simulink model "ObstacleDetectionDemo"  (R2020a)
settings: Solver=FixedStepDiscrete  StartTime=0.0  StopTime=inf  FixedStep=params.Ts  RelTol=1e-3  EnableMultiTasking=on
PreLoadFcn:
  | params = controlParamsGazebo;
  | 
  | rosshutdown;
  | loadIpAddresses;
  | rosinit(gazeboIp);
model workspace (MAT data in the model file):
  SL_ROS_VariableLengthArrays_MaxSizes.CommonInfo.ArrayTruncateAction = 'EmitWarning'
  SL_ROS_VariableLengthArrays_MaxSizes.MsgTypeMap = containers.Map
  SL_ROS_VariableLengthArrays_MaxSizes.MsgTypeMap.serialization.keys = {'sensor_msgs/CompressedImage', 'sensor_msgs/Image'}
  SL_ROS_VariableLengthArrays_MaxSizes.MsgTypeMap.serialization.values{1}(1).PropertyName = 'Data'
  SL_ROS_VariableLengthArrays_MaxSizes.MsgTypeMap.serialization.values{1}(1).DataType = 'uint8'
  SL_ROS_VariableLengthArrays_MaxSizes.MsgTypeMap.serialization.values{1}(1).MaxLength = 26264
  SL_ROS_VariableLengthArrays_MaxSizes.MsgTypeMap.serialization.values{1}(2).PropertyName = 'Format'
  SL_ROS_VariableLengthArrays_MaxSizes.MsgTypeMap.serialization.values{1}(2).DataType = 'uint8'
  SL_ROS_VariableLengthArrays_MaxSizes.MsgTypeMap.serialization.values{1}(2).MaxLength = 128
  SL_ROS_VariableLengthArrays_MaxSizes.MsgTypeMap.serialization.values{2}(1).PropertyName = 'Data'
  SL_ROS_VariableLengthArrays_MaxSizes.MsgTypeMap.serialization.values{2}(1).DataType = 'uint8'
  SL_ROS_VariableLengthArrays_MaxSizes.MsgTypeMap.serialization.values{2}(1).MaxLength = 921600
  SL_ROS_VariableLengthArrays_MaxSizes.MsgTypeMap.serialization.values{2}(2).PropertyName = 'Encoding'
  SL_ROS_VariableLengthArrays_MaxSizes.MsgTypeMap.serialization.values{2}(2).DataType = 'uint8'
  SL_ROS_VariableLengthArrays_MaxSizes.MsgTypeMap.serialization.values{2}(2).MaxLength = 128
  SL_ROS_VariableLengthArrays_MaxSizes.MsgTypeMap.serialization.uniformity = 0
  SL_ROS_VariableLengthArrays_MaxSizes.MsgTypeMap.serialization.keyType = 'char'
  SL_ROS_VariableLengthArrays_MaxSizes.MsgTypeMap.serialization.valueType = 'any'
libraries: robotlib x11
settings Model: Creator=scastro  LastModifiedBy=shiva
settings SolverCC: PositivePriorityOrder=on
settings DataIOCC: ReturnWorkspaceOutputs=off
settings OptimizationCC: PassReuseOutputArgsAs=Individual arguments  MaxStackSize=64  EfficientTunableParamExpr=on
settings DebuggingCC: ParameterTunabilityLossMsg=error  ArithmeticOperatorsInVariantConditions=warning
settings HardwareCC: ProdBitPerLong=64  ProdHWDeviceType=Intel->x86-64 (Linux 64)  UseEmbeddedCoderFeatures=off
settings SFSimCC: SimUseLocalCustomCode=off  CustomCodeUndefinedFunction=UseInterfaceOnly
settings RTWCC: SystemTargetFile=ert.tlc  HardwareBoard=Robot Operating System (ROS)  TemplateMakefile=ert_default_tmf  GenerateReport=on  RTWUseLocalCustomCode=off  Toolchain=Catkin  IncludeHyperlinkInReport=on  LaunchReport=on  TargetLang=C++  GenerateTraceInfo=on  GenerateTraceReport=on  GenerateTraceReportSl=on  GenerateTraceReportSf=on  GenerateTraceReportEml=on
settings CodeAppCC: ForceParamTrailComments=on  IgnoreCustomStorageClasses=off  OperatorAnnotations=on  SimulinkDataObjDesc=on  SFDataObjDesc=on  MATLABFcnDesc=on  InsertBlockDesc=on  StateflowObjectComments=on  MATLABSourceComments=on
settings ERTTargetCC: SupportNonInlinedSFcns=on  SupportVariableSizeSignals=on

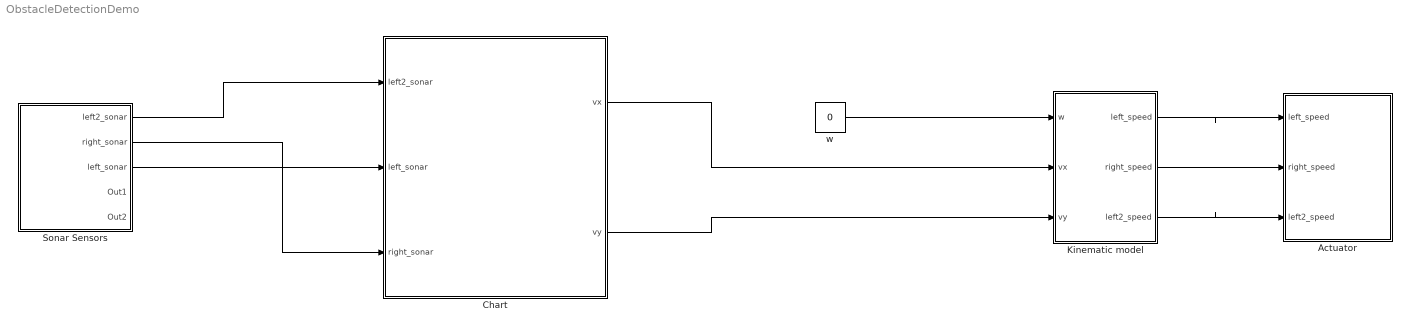
== system ObstacleDetectionDemo ==
  Actuator : Subsystem
  Chart : Stateflow chart  TreatAsAtomicUnit=on
  Kinematic model : Subsystem
  Sonar Sensors : Subsystem
  w : Constant  Value=0
  wires:
  w/1 -> Kinematic model/1(w)
  Chart/1(vx) -> Kinematic model/2(vx)
  Chart/2(vy) -> Kinematic model/3(vy)
  Kinematic model/1(left_speed) -> Actuator/1(left_speed)
  Kinematic model/2(right_speed) -> Actuator/2(right_speed)
  Kinematic model/3(left2_speed) -> Actuator/3(left2_speed)
  Sonar Sensors/1(left2_sonar) -> Chart/1(left2_sonar)
  Sonar Sensors/2(right_sonar) -> Chart/3(right_sonar)
  Sonar Sensors/3(left_sonar) -> Chart/2(left_sonar)

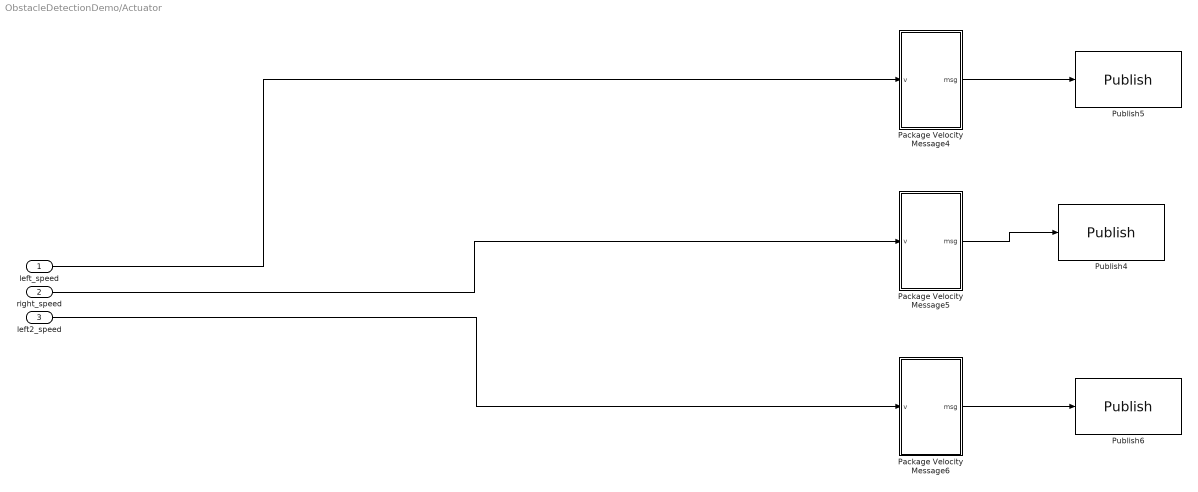
== system ObstacleDetectionDemo/Actuator ==
  left_speed : Inport
  right_speed : Inport  Port=2
  left2_speed : Inport  Port=3
  Package Velocity Message4 : Subsystem
  Package Velocity Message5 : Subsystem
  Package Velocity Message6 : Subsystem
  Publish4 : robotlib/Publish  topicSource=Select from ROS network  topic=/robot/right_joint_velocity_controller/command  messageType=std_msgs/Float64  messageQueueLength=1
  Publish5 : robotlib/Publish  topicSource=Select from ROS network  topic=/robot/left_joint_velocity_controller/command  messageType=std_msgs/Float64  messageQueueLength=1
  Publish6 : robotlib/Publish  topicSource=Select from ROS network  topic=/robot/left2_joint_velocity_controller/command  messageType=std_msgs/Float64  messageQueueLength=1
  wires:
  left_speed/1 -> Package Velocity Message4/1(v)
  Package Velocity Message6/1(msg) -> Publish6/1
  right_speed/1 -> Package Velocity Message5/1(v)
  Package Velocity Message4/1(msg) -> Publish5/1
  Package Velocity Message5/1(msg) -> Publish4/1
  left2_speed/1 -> Package Velocity Message6/1(v)

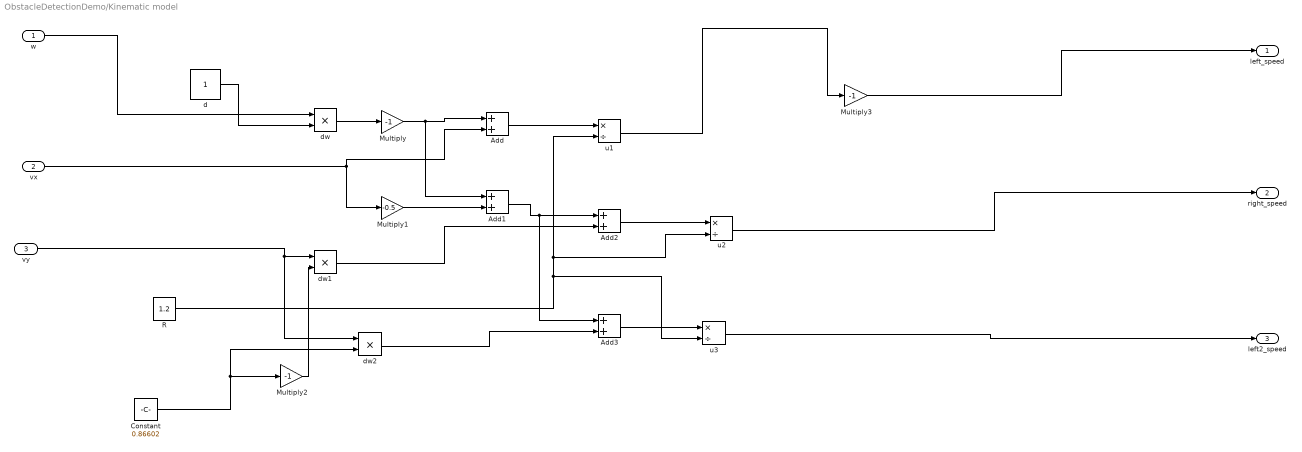
== system ObstacleDetectionDemo/Kinematic model ==
  w : Inport
  vx : Inport  Port=2
  vy : Inport  Port=3
  Add{,1..3} (4 alike) : Sum
  Constant : Constant  Value=0.86602
  Multiply : Gain  Gain=-1
  Multiply1 : Gain  Gain=-0.5
  Multiply2 : Gain  Gain=-1
  Multiply3 : Gain  Gain=-1
  R : Constant  Value=1.2
  d : Constant  VectorParams1D=off  SampleTime=-1
  dw : Product
  dw1 : Product
  dw2 : Product
  u1 : Product  Inputs=*/
  u2 : Product  Inputs=*/
  u3 : Product  Inputs=*/
  left_speed : Outport
  right_speed : Outport  Port=2
  left2_speed : Outport  Port=3
  wires:
  Multiply/1 -> Add1/1, Add/1
  Add/1 -> u1/1
  Multiply3/1 -> left_speed/1
  dw1/1 -> Add2/2
  w/1 -> dw/1
  Multiply2/1 -> dw1/2
  Add1/1 -> Add3/1, Add2/1
  Constant/1 -> dw2/2, Multiply2/1
  u3/1 -> left2_speed/1
  vy/1 -> dw2/1, dw1/1
  dw2/1 -> Add3/2
  d/1 -> dw/2
  u2/1 -> right_speed/1
  R/1 -> u3/2, u2/2, u1/2
  Add3/1 -> u3/1
  dw/1 -> Multiply/1
  vx/1 -> Add/2, Multiply1/1
  u1/1 -> Multiply3/1
  Add2/1 -> u2/1
  Multiply1/1 -> Add1/2

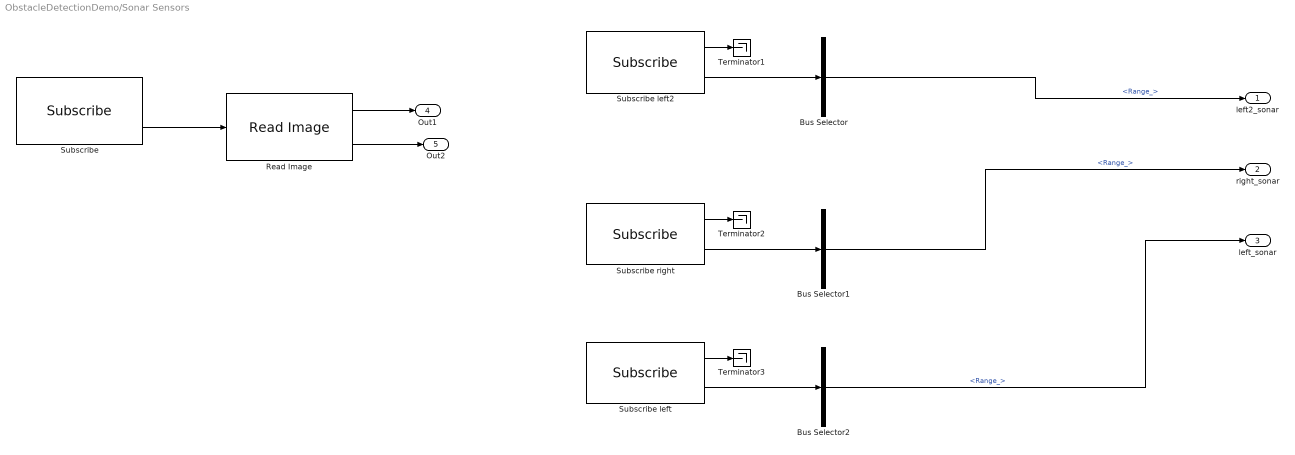
== system ObstacleDetectionDemo/Sonar Sensors ==
  Bus Selector : BusSelector  OutputSignals=Range_
  Bus Selector1 : BusSelector  OutputSignals=Range_
  Bus Selector2 : BusSelector  OutputSignals=Range_
  Read Image : robotlib/Read Image  MaximumImageSize=[1020, 1020]  ImageEncoding=rgb8  ShowAlphaOutput=off  ShowErrorCodeOutput=on  VariableSizeOutputs=off
      settings: SourceProductBaseCode=RR
  Subscribe : robotlib/Subscribe  topicSource=Select from ROS network  topic=/robot_sensor/camera/image_raw/compressed  messageType=sensor_msgs/CompressedImage  sampleTime=-1  messageQueueLength=1
  Subscribe left : robotlib/Subscribe  topicSource=Select from ROS network  topic=/sonar_sonar_link_3  messageType=sensor_msgs/Range  sampleTime=-1  messageQueueLength=1
  Subscribe left2 : robotlib/Subscribe  topicSource=Select from ROS network  topic=/sonar_sonar_link_1  messageType=sensor_msgs/Range  sampleTime=-1  messageQueueLength=1
  Subscribe right : robotlib/Subscribe  topicSource=Select from ROS network  topic=/sonar_sonar_link_2  messageType=sensor_msgs/Range  sampleTime=-1  messageQueueLength=1
  Terminator1 : Terminator
  Terminator2 : Terminator
  Terminator3 : Terminator
  left2_sonar : Outport
  right_sonar : Outport  Port=2
  left_sonar : Outport  Port=3
  Out1 : Outport  Port=4
  Out2 : Outport  Port=5
  wires:
  Bus Selector1/1 -> right_sonar/1  "<Range_>"
  Subscribe left/1 -> Terminator3/1
  Subscribe left/2 -> Bus Selector2/1
  Subscribe left2/1 -> Terminator1/1
  Subscribe right/1 -> Terminator2/1
  Bus Selector/1 -> left2_sonar/1  "<Range_>"
  Subscribe right/2 -> Bus Selector1/1
  Subscribe left2/2 -> Bus Selector/1
  Bus Selector2/1 -> left_sonar/1  "<Range_>"
  Subscribe/2 -> Read Image/1
  Read Image/1 -> Out1/1
  Read Image/2 -> Out2/1

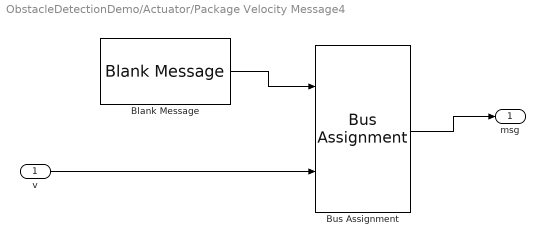
== system ObstacleDetectionDemo/Actuator/Package Velocity Message4 ==
  v : Inport
  Blank Message : robotlib/Blank Message  messageClass=Message  entityType=std_msgs/Float64  messageType=std_msgs/Float64  SampleTime=inf
  Bus Assignment : BusAssignment  AssignedSignals=Data
  msg : Outport  VectorParamsAs1DForOutWhenUnconnected=off
  wires:
  Blank Message/1 -> Bus Assignment/1
  Bus Assignment/1 -> msg/1
  v/1 -> Bus Assignment/2

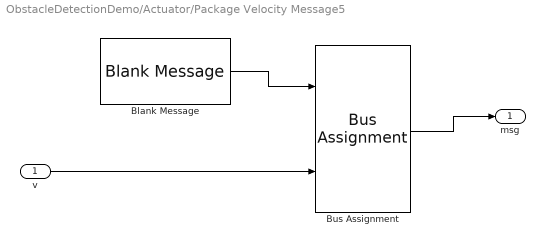
== system ObstacleDetectionDemo/Actuator/Package Velocity Message5 ==
  v : Inport
  Blank Message : robotlib/Blank Message  messageClass=Message  entityType=std_msgs/Float64  messageType=std_msgs/Float64  SampleTime=inf
  Bus Assignment : BusAssignment  AssignedSignals=Data
  msg : Outport  VectorParamsAs1DForOutWhenUnconnected=off
  wires:
  Blank Message/1 -> Bus Assignment/1
  Bus Assignment/1 -> msg/1
  v/1 -> Bus Assignment/2

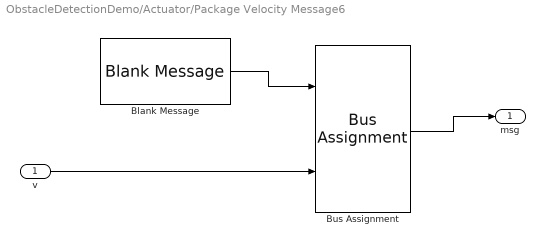
== system ObstacleDetectionDemo/Actuator/Package Velocity Message6 ==
  v : Inport
  Blank Message : robotlib/Blank Message  messageClass=Message  entityType=std_msgs/Float64  messageType=std_msgs/Float64  SampleTime=inf
  Bus Assignment : BusAssignment  AssignedSignals=Data
  msg : Outport  VectorParamsAs1DForOutWhenUnconnected=off
  wires:
  Blank Message/1 -> Bus Assignment/1
  Bus Assignment/1 -> msg/1
  v/1 -> Bus Assignment/2

== stateflow chart ObstacleDetectionDemo/Chart ==
  state left2_obs
    entry:
    vx = speed_gain;
    vy = 0.57735026919 *speed_gain;
  state left_left2_obs
    entry:
    vx = speed_gain;
    vy = -0.57735026919 *speed_gain;
  state left_right_obs
    entry:
    vy = -0.57735026919 * speed_gain ;
    vx = -1*speed_gain;
  state INIT
  state right_obs
    entry:
    vx = -1*speed_gain;
    vy = 0.57735026919 *speed_gain;
  state right_left2_obs
    entry:
    vx = 0;
    vy = speed_gain;
  state left_obs
    entry:
    vx = 0;
    vy =-1*speed_gain;
  INIT -> left2_obs [order 1] : [left2_sonar >= 1 && left_sonar < 1 && right_sonar <1 ]
  left2_obs -> INIT : [after(1,msec)]
  left_left2_obs -> INIT : [after(1,msec)]
  INIT -> left_left2_obs [order 5] : [left2_sonar >= 1 && left_sonar >= 1 && right_sonar <1 ]
  INIT -> left_right_obs [order 6] : [left2_sonar < 1 && left_sonar >= 1 && right_sonar >=1 ]
  (default) -> INIT
  right_obs -> INIT : [after(1,msec)]
  left_right_obs -> INIT : [after(1,msec)]
  INIT -> right_left2_obs [order 4] : [left2_sonar >= 1 && left_sonar < 1 && right_sonar >=1 ]
  INIT -> right_obs [order 3] : [left2_sonar < 1 && left_sonar < 1 && right_sonar >1 ]
  right_left2_obs -> INIT : [after(1,msec)]
  INIT -> left_obs [order 2] : [left2_sonar < 1 && left_sonar >= 1 && right_sonar <1 ]
  left_obs -> INIT : [after(1,msec)]
  data: left2_sonar input; vx output; vy output =10; speed_gain local =7; left_sonar input; right_sonar input
